simulink model "socket_test"  (Simulink 9.2)
settings: Solver=FixedStepDiscrete  StartTime=0.0  StopTime=Inf  RelTol=1e-3  EnableMultiTasking=on
libraries: rpi_blkst x2
settings Model: Creator=jacques  LastModifiedBy=jacques  SimulationMode=external
settings OptimizationCC: ExpressionDepthLimit=2147483647  LifeSpan=1
settings DebuggingCC: SolverPrmCheckMsg=warning
settings HardwareCC: ProdLargestAtomicInteger=Long  ProdLargestAtomicFloat=Double  ProdIntDivRoundTo=Zero  ProdEndianess=LittleEndian  ProdHWDeviceType=ARM Compatible->ARM Cortex
settings SFSimCC: MATLABDynamicMemAlloc=off
settings RTWCC: SystemTargetFile=ert_rpi.tlc  TemplateMakefile=ert_rpi.tmf  PostCodeGenCommand=postGenFunc(buildInfo)  Description=RTW Embedded Coder RPI target
settings CodeAppCC: IgnoreCustomStorageClasses=off  CustomSymbolStrType=$N$R$M  InternalIdentifier=Classic
settings STFCustomTargetCC: ModelReferenceCompliant=off  CombineOutputUpdateFcns=on  ERTCustomFileBanners=on  SupportNonInlinedSFcns=off  RemoveResetFunc=on  MATLABClassNameForMDSCustomization=Simulink.SoftwareTarget.ERTCustomization  GRTInterface=off  SystemTargetFile=ert_rpi.tlc
settings ERTTargetCC: MultiwordLength=2048  ModelReferenceCompliant=off  ParMdlRefBuildCompliant=off  CompOptLevelCompliant=off  ConcurrentExecutionCompliant=off  SupportContinuousTime=on  ModelStepFunctionPrototypeControlCompliant=off  CPPClassGenCompliant=off  UseToolchainInfoCompliant=off  ExtMode=on  ExtModeMexArgs='10.211.55.4'  ERTCustomFileTemplate=ert_rpi_file_process.tlc  ConvertIfToSwitch=off  SuppressUnreachableDefaultCases=off

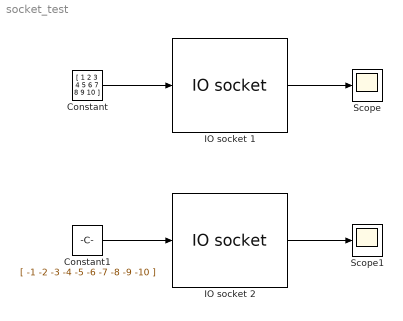
== system socket_test ==
  Constant : Constant  Value=[ 1 2 3 4 5 6 7 8 9 10 ]  SampleTime=0.01
  Constant1 : Constant  Value=[ -1 -2 -3 -4 -5 -6 -7 -8 -9 -10 ]  SampleTime=0.01
  IO socket 1 : rpi_blkst/IO socket  rpi_mask_Ts=0.01  rpi_mask_ip1=10  rpi_mask_ip2=211  rpi_mask_ip3=55  rpi_mask_ip4=4
      settings: SourceProductName=RPI Blockset
  IO socket 2 : rpi_blkst/IO socket  rpi_mask_Ts=0.01  rpi_mask_ip1=10  rpi_mask_ip2=0  rpi_mask_ip3=1  rpi_mask_ip4=3
      settings: SourceProductName=RPI Blockset
  Scope : Scope
  Scope1 : Scope
  wires:
  IO socket 1/1 -> Scope/1
  Constant/1 -> IO socket 1/1
  IO socket 2/1 -> Scope1/1
  Constant1/1 -> IO socket 2/1
